simulink model "MotorTest"  (R2021a)
settings: Solver=FixedStepAuto  StartTime=0.0  StopTime=50.0  FixedStep=0.001  RelTol=1e-3  EnableMultiTasking=on
libraries: arduinolib x3, simulink x2
settings Model: SILPILModeSetting=veronly  ExtModeTrigDuration=2  Creator=drak0  LastModifiedBy=drak0
settings SolverCC: AutoInsertRateTranBlk=on
settings OptimizationCC: EnhancedBackFolding=on  PassReuseOutputArgsAs=Individual arguments  ZeroExternalMemoryAtStartup=off  ZeroInternalMemoryAtStartup=off  MaxStackSize=64  OptimizeBlockOrder=speed  DifferentSizesBufferReuse=on  OptimizationCustomize=off  EfficientTunableParamExpr=on
settings DebuggingCC: ParameterTunabilityLossMsg=error
settings HardwareCC: ProdBitPerInt=16  ProdBitPerPointer=16  ProdBitPerSizeT=16  ProdBitPerPtrDiffT=16  ProdLargestAtomicFloat=None  ProdWordSize=8  ProdHWDeviceType=Atmel->AVR  UseEmbeddedCoderFeatures=off  UseSimulinkCoderFeatures=off
settings SFSimCC: MATLABDynamicMemAlloc=off
settings RTWCC: SystemTargetFile=ert.tlc  HardwareBoard=Arduino Mega 2560  TemplateMakefile=ert_default_tmf  Toolchain=Arduino AVR  BuildConfiguration=Faster Runs
settings CodeAppCC: ForceParamTrailComments=on  IgnoreCustomStorageClasses=off  OperatorAnnotations=on  SimulinkDataObjDesc=on  SFDataObjDesc=on  InsertBlockDesc=on
settings ERTTargetCC: SupportContinuousTime=on  SupportNonInlinedSFcns=on  SupportVariableSizeSignals=on  ExtModeStaticAllocSize=2048

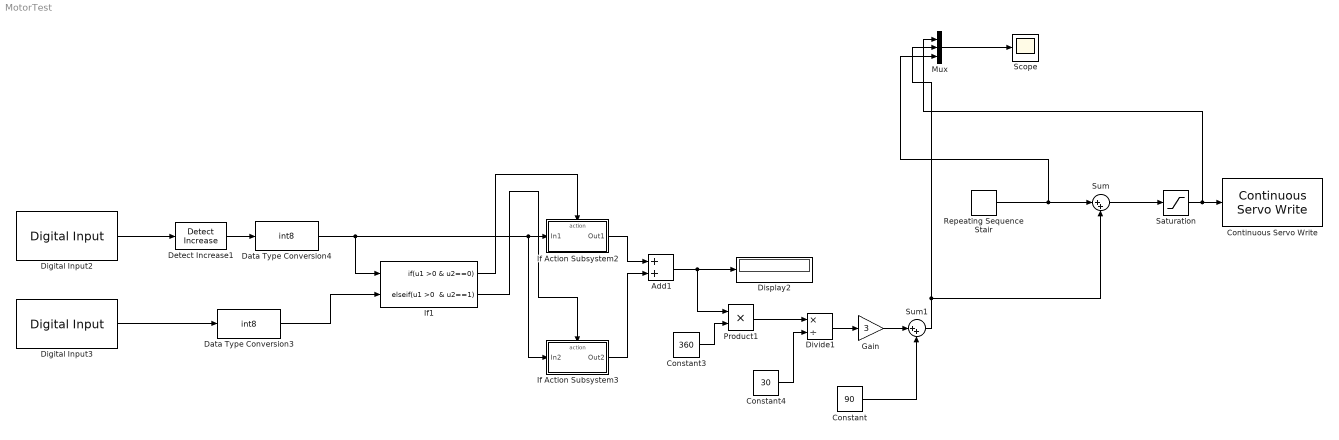
== system MotorTest ==
  Add1 : Sum
  Constant : Constant  Value=90
  Constant3 : Constant  Value=360
  Constant4 : Constant  Value=30
  Continuous Servo Write : arduinolib/Continuous Servo Write  pinNumber=10  ServoIndex=0  blockPlatform=ARDUINO
      settings: SourceProductBaseCode=ARDUINO
  Data Type Conversion3 : DataTypeConversion  OutDataTypeStr=int8
  Data Type Conversion4 : DataTypeConversion  OutDataTypeStr=int8
  Detect Increase1 : simulink/Logic and Bit Operations/Detect Increase  vinit=0.0  OutDataTypeStr=boolean
  Digital Input2 : arduinolib/Digital Input  pinNumber=2  mode=Default  Direction=input  SampleTime=0.001  blockPlatform=arduino
  Digital Input3 : arduinolib/Digital Input  pinNumber=3  mode=Default  Direction=input  SampleTime=0.001  blockPlatform=arduino
  Display2 : Display
  Divide1 : Product  Inputs=*/
  Gain : Gain  Gain=3
  If Action Subsystem2 : Subsystem  TreatAsAtomicUnit=on
  If Action Subsystem3 : Subsystem  TreatAsAtomicUnit=on
  If1 : If  NumInputs=2  IfExpression=u1 >0 & u2==0  ElseIfExpressions="u1 >0  & u2==1"  ShowElse=off
  Mux : Mux  Inputs=3
  Product1 : Product
  Repeating Sequence Stair : simulink/Sources/Repeating Sequence Stair  OutValues=[0:5:180 180:-5:0].'  tsamp=0.1  OutMin=[]  OutMax=[]  OutDataTypeStr=double  OutputDataTypeScalingMode=double  OutDataType=fixdt(0,8)  ConRadixGroup=Best Precision: Vector-wise  OutScaling=2^-12
  Saturation : Saturate  UpperLimit=180  LowerLimit=0
  Scope : Scope
  Sum : Sum  Inputs=|++
  Sum1 : Sum  Inputs=|++
  wires:
  Digital Input2/1 -> Detect Increase1/1
  If1/2 -> If Action Subsystem3/Action
  Data Type Conversion4/1 -> If Action Subsystem3/1(In2), If Action Subsystem2/1(In1), If1/1
  Digital Input3/1 -> Data Type Conversion3/1
  Product1/1 -> Divide1/1
  If1/1 -> If Action Subsystem2/Action
  If Action Subsystem2/1(Out1) -> Add1/1
  Constant3/1 -> Product1/2
  Detect Increase1/1 -> Data Type Conversion4/1
  Constant4/1 -> Divide1/2
  Add1/1 -> Product1/1, Display2/1
  Data Type Conversion3/1 -> If1/2
  If Action Subsystem3/1(Out2) -> Add1/2
  Mux/1 -> Scope/1
  Repeating Sequence Stair/1 -> Mux/3, Sum/1
  Sum/1 -> Saturation/1
  Divide1/1 -> Gain/1
  Saturation/1 -> Mux/1, Continuous Servo Write/1
  Constant/1 -> Sum1/2
  Gain/1 -> Sum1/1
  Sum1/1 -> Sum/2, Mux/2

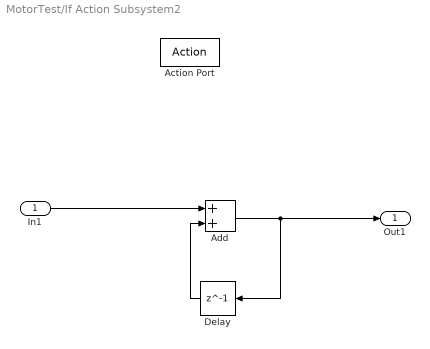
== system MotorTest/If Action Subsystem2 ==
  In1 : Inport
  Action Port : ActionPort  ActionPortLabel=if(u1 >0 & u2==0)
  Add : Sum
  Delay : Delay  DelayLength=1  InitialCondition=0
  Out1 : Outport
  wires:
  In1/1 -> Add/1
  Add/1 -> Delay/1, Out1/1
  Delay/1 -> Add/2

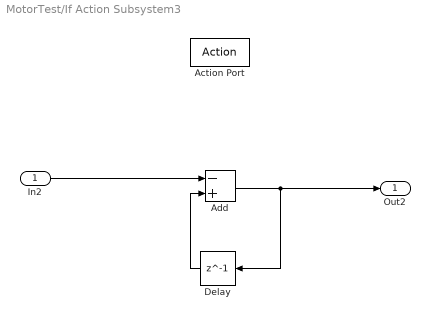
== system MotorTest/If Action Subsystem3 ==
  In2 : Inport
  Action Port : ActionPort  ActionPortLabel="elseif( u1 >0  & u2==1)"
  Add : Sum  Inputs=-+
  Delay : Delay  DelayLength=1  InitialCondition=0
  Out2 : Outport
  wires:
  In2/1 -> Add/1
  Delay/1 -> Add/2
  Add/1 -> Delay/1, Out2/1
